simulink model "Power_Generator_Working"  (R2019b)
settings: Solver=ode23tb  StartTime=0.0  StopTime=inf  RelTol=5e-3
model workspace (MAT data in the model file):
  PLC_IP_Address = 'localhost'
libraries: dspnetwork x28, powerlib x8, sps_avr x7, simulink x3, dspstat3 x2
Description:
  | Copyright 2008-2019 The MathWorks, Inc.
settings Model: FPTRunName=Active  EnablePacing=on  PacingRate=0.100000  ExtModeTrigMode=oneshot  ExtModeArmWhenConnect=off  ExtModeAutoUpdateStatusClock=off  Creator=MathWorks  LastModifiedBy=Barata
settings SolverCC: ZeroCrossAlgorithm=Adaptive
settings DataIOCC: SaveFormat=Array  SignalLoggingSaveFormat=ModelDataLogs  ReturnWorkspaceOutputs=off  SignalLoggingName=sigsOut  OutputTimes=[0:1/20:10]
settings OptimizationCC: BlockReduction=off  BooleanDataType=off  ExpressionDepthLimit=2147483647  InitFltsAndDblsToZero=on  EfficientMapNaN2IntZero=off  LifeSpan=inf
settings DebuggingCC: UnderspecifiedInitializationDetection=Classic  MergeDetectMultiDrivingBlocksExec=none  CheckExecutionContextPreStartOutputMsg=on  CheckExecutionContextRuntimeOutputMsg=on  SignalResolutionControl=TryResolveAllWithWarning  IgnoredZcDiagnostic=none  MultiTaskDSMMsg=warning  MultiTaskCondExecSysMsg=none  SigSpecEnsureSampleTimeMsg=none  FcnCallInpInsideContextMsg=warning  UnconnectedInputMsg=none  UnconnectedOutputMsg=none  UnconnectedLineMsg=none  StateNameClashWarn=warning  SFUnexpectedBacktrackingDiag=warning  SFNoUnconditionalDefaultTransitionDiag=warning  SFExecutionAtInitializationDiag=none  ArithmeticOperatorsInVariantConditions=warning
settings HardwareCC: ProdBitPerPointer=32  ProdBitPerSizeT=32  ProdBitPerPtrDiffT=32  ProdLargestAtomicFloat=None  ProdIntDivRoundTo=Undefined  ProdEndianess=Unspecified  ProdWordSize=32  ProdHWDeviceType=Specified  TargetUnknown=on
settings ModelReferenceCC: PropagateSignalLabelsOutOfModel=off
settings SFSimCC: SimUseLocalCustomCode=off  CustomCodeUndefinedFunction=UseInterfaceOnly
settings RTWCC: RTWUseLocalCustomCode=off
settings CodeAppCC: StateflowObjectComments=on
settings GRTTargetCC: TargetFcnLib=ansi_tfl_tmw.mat  TargetLangStandard=C89/C90 (ANSI)  GeneratePreprocessorConditionals=Disable all  CombineOutputUpdateFcns=off  GRTInterface=on
settings ConfigComp: CovMetricSettings=dw  CovHtmlReporting=on  CovSaveCumulativeToWorkspaceVar=on  CovSaveSingleToWorkspaceVar=on  CovExternalEMLEnable=off  CovSFcnEnable=off
settings SimscapeCC: SimscapeNormalizeSystem=off

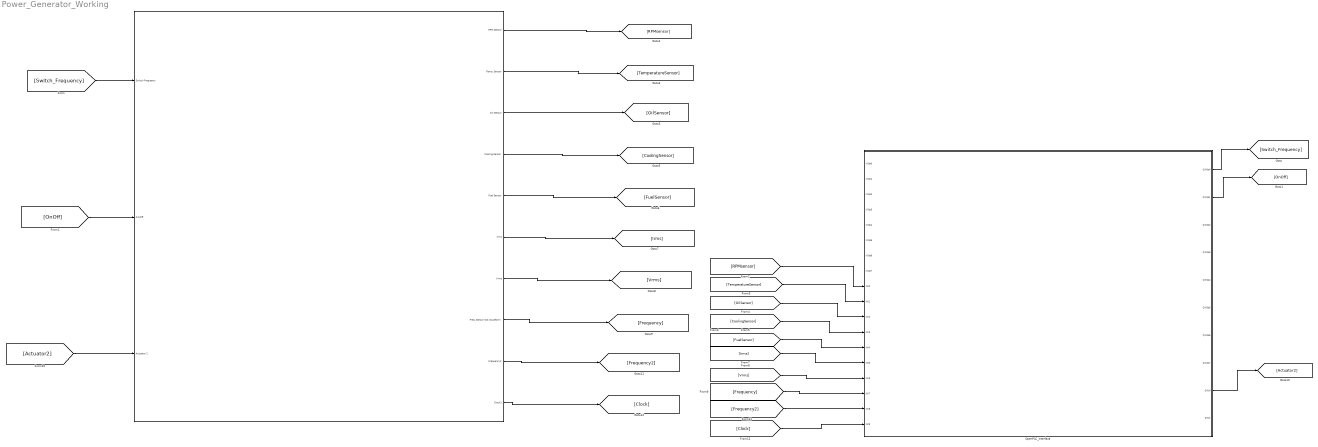
== system Power_Generator_Working ==
  " " : Subsystem
  OpenPLC_Interface : Subsystem
  wires:
  OpenPLC_Interface/2(QX0p1) -> [OnOff]
  [RPMsensor] -> OpenPLC_Interface/9(IW0)
  OpenPLC_Interface/1(QX0p0) -> [Switch_Frequency]
  [TemperatureSensor] -> OpenPLC_Interface/10(IW1)
  [OilSensor] -> OpenPLC_Interface/11(IW2)
  [CoolingSensor] -> OpenPLC_Interface/12(IW3)
  [FuelSensor] -> OpenPLC_Interface/13(IW4)
  [Irms] -> OpenPLC_Interface/14(IW5)
  [Vrms] -> OpenPLC_Interface/15(IW6)
  " "/1(RPM Sensor) -> [RPMsensor]
  " "/2("Temp. Sensor ") -> [TemperatureSensor]
  " "/4(Cooling Sensor) -> [CoolingSensor]
  " "/6(Irms) -> [Irms]
  " "/7(Vrms) -> [Vrms]
  " "/8("Freq. Sensor Not Waveform ") -> [Frequency]
  [Switch_Frequency] -> " "/1(Switch Frequency)
  [OnOff] -> " "/2(On/Off)
  [Frequency] -> OpenPLC_Interface/16(IW7)
  " "/3(Oil Sensor) -> [OilSensor]
  " "/5(Fuel Sensor) -> [FuelSensor]
  [Actuator2] -> " "/3(Actuator 2)
  OpenPLC_Interface/9(QW0) -> [Actuator2]
  " "/9(" Frequency2") -> [Frequency2]
  [Frequency2] -> OpenPLC_Interface/17(IW8)
  " "/10(Clock1) -> [Clock]
  [Clock] -> OpenPLC_Interface/18(IW9)

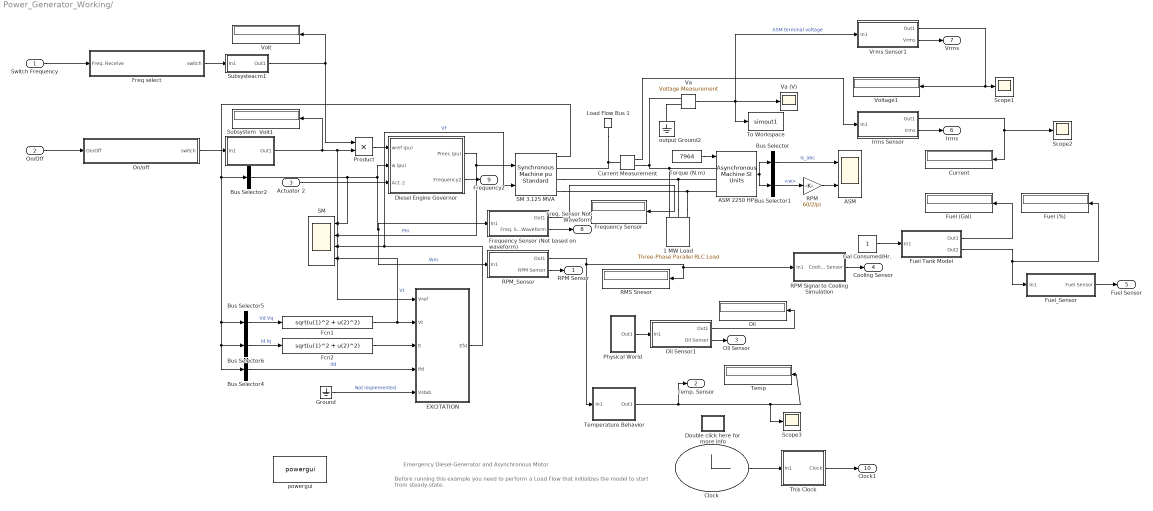
== system Power_Generator_Working/  ==
  note: Before running this example you need to perform a Load Flow that
      | initializes the model to start from steady-state.
  note: Emergency Diesel-Generator and Asynchronous Motor
  Switch Frequency : Inport
  On/Off : Inport  Port=2
  Actuator 2 : Inport  Port=3
  1 MW Load : powerlib/Elements/Three-Phase Parallel RLC Load  LConnTagsString=A|B|C  Configuration=Y (grounded)  NominalVoltage=2400  Vabc=[1e3 1e3 1e3]  Vabcp=[1e3 1e3 1e3]  NominalFrequency=60  UnbalancedPower=off  ActivePower=1e+006  InductivePower=0  CapacitivePower=0  Pabc=[10e3 9e3 11e3]  QLabc=[100 90 110]  QCabc=[100 90 110]  Pabcp=[10e3 9e3 11e3]  QLabcp=[100 90 110]  QCabcp=[100 90 110]  Measurements=None  LoadType=constant Z
      settings: SourceProductName=Simscape Electrical
  ASM : Scope  NumInputPorts=2
  ASM 2250 HP : powerlib/Machines/Asynchronous Machine SI Units  RotorType=Squirrel-cage  PresetModel=No  MechanicalLoad=Torque Tm  ShowDetailedParameters=on  ReferenceFrame=Rotor  Units=SI  MeasurementBus=on  NominalParameters=[ 2250*746, 2400, 60 ]  Stator=[ 0.029 0.226/377]  Rotor=[ 0.022 0.226/377]  Cage1=[ 0.022 0.226/377]  Cage2=[ 0.022 0.226/377]  Lm=13.04/377  Mechanical=[ 63.87 0 2]  PolePairs=2  InitialConditions=[0 0 0 0 0 0 0 0]  SimulateSaturation=off  Saturation=[14.03593122, 27.81365428, 53.79336849, 72.68890987, 97.98006896, 148.6815601, 215.7428561, 302.9841135, 428.7778367 ; 230, 322, 414, 460, 506, 552, 598, 644, 690]  LoadFlowParameters=1492000  TsPowergui=0  TsBlock=-1  IterativeModel=Trapezoidal non iterative  IterativeDiscreteModel=Trapezoidal non iterative  Pmec=1.492e+006
      settings: SourceProductName=Simscape Electrical
  Bus Selector : BusSelector  OutputSignals=ias,ibs,ics  OutputAsBus=on
  Bus Selector1 : BusSelector  OutputSignals=w
  Bus Selector2 : BusSelector  OutputSignals="Mechanical.Rotor speed  wm  (pu)"  OutputAsBus=on
  Bus Selector4 : BusSelector  OutputSignals="dq0 components.Field current  ifd (pu)"  OutputAsBus=on
  Bus Selector5 : BusSelector  OutputSignals="dq0 components.Stator voltage  vd (pu),dq0 components.Stator voltage  vq (pu)"  OutputAsBus=on
  Bus Selector6 : BusSelector  OutputSignals="dq0 components.Stator current  id (pu),dq0 components.Stator current  iq (pu)"  OutputAsBus=on
  Clock : Clock
  Current : Display
  Current Measurement : powerlib/Measurements/Current Measurement  PhasorSimulation=off  OutputType=Complex  PSBequivalent=0
      settings: SourceProductName=Simscape Electrical
  Diesel Engine Governor : Subsystem  AncestorBlock=spsDieselMotorModel/Diesel Engine Governor  mask(Diesel Engine & Governor){K=40, Tr=[0.01 0.02 0.2], Ta=[0.25 0.009 0.0384], Tlim=[0 1.1], Td=0.024, Pm0=0}
      mask prompts: K "Regulator gain K:"; Tr "Regulator time constants [T1 T2 T3 ] (s) :"; Ta "Actuator time constants [T4 T5 T6] (s) :"; Tlim "Torque limits [Tmin Tmax] (pu) :"; Td "Engine time delay Td (s) :"; Pm0 "Initial value of mechanical power  Pm0 (pu) :"
      mask help:
      | This block implements a diesel engine and governor system. The first input is the reference speed and the second input is the measured speed. The output is the diesel engine mechanical power. The motor inertia should be combined with the generator inertia.
      |
      | The model consist of a regulator represented by the following transfer function:
      |
      |      Hc = K.(1+T3.s)/(1+T1.s+T1.T2.s^2)
      |
      | The trotte actuator is implemented as :
      |
      |      Ha =  (1+T4.s) / [ (s (1+T5.s)(1+T6.s) ]
      |
      | The motor engine is represented by a Time delay Td function.
      mask Help:
      | This block implements a diesel engine and governor system. The first input is the reference speed and the second input is the measured speed. The output is the diesel engine mechanical power. The motor inertia should be combined with the generator inertia.
      | 
      | The model consist of a regulator represented by the following transfer function:
      | 
      |      Hc = K.(1+T3.s)/(1+T1.s+T1.T2.s^2)
      | 
      | The trotte actuator is implemented as :
      | 
      |      Ha =  (1+T4.s) / [ (s (1+T5.s)(1+T6.s) ]
      | 
      | The motor engine is represented by a Time delay Td function.
  Double click here for more info : Subsystem
      settings: OpenFcn=showdemo(bdroot(gcb))
      mask Display: disp('?')
  EXCITATION : Subsystem  VariantControlMode=Label  Variant=on  LabelModeActiveChoice=Variant1
      settings: AttributesFormatString=%<BlockChoice>
  Fcn1 : Fcn  Expr=sqrt(u(1)^2 + u(2)^2)
  Fcn2 : Fcn  Expr=sqrt(u(1)^2 + u(2)^2)
  Freq select : Subsystem
  Frequency Sensor : Display
  Frequency Sensor (Not based on waveform) : Subsystem
  Fuel (%) : Display
  Fuel (Gal) : Display
  Fuel Tank Model : Subsystem
  Fuel_Sensor : Subsystem
  "Gal Consumed/Hr. " : Constant
  Ground : Ground
  Irms Sensor : Subsystem
  Load Flow Bus 1 : powerlib/Measurements/Load Flow Bus  LConnTagsString=a  Phases=single  Connectors=on one side  ID=B2  Vbase=2.4e3  Vref=1  Vangle=0  VLF=1  VLFb=1  VLFc=1  angleLF=-31.89  angleLFb=0  angleLFc=0
      settings: AttributesFormatString=%<ID>\n%<Vbase>V\n%<VLF>pu\n%<angleLF>deg.  SourceProductName=Simscape Electrical
  Oil : Display
  Oil Sensor1 : Subsystem
  On/off : Subsystem
  Physical World : Subsystem
  Product : Product
  RMS Snesor : Display
  RPM : Gain  Gain=60/2/pi  SaturateOnIntegerOverflow=on  OutDataTypeStr=Inherit: Same as input  ParamDataTypeStr=Inherit: Same as input
  RPM Signal to Cooling Simulation : Subsystem
  RPM_Sensor : Subsystem
  SM : Scope  NumInputPorts=4
  SM 3.125 MVA : powerlib/Machines/Synchronous Machine pu Standard  PresetModel=No  MechanicalLoad=Mechanical power Pm  ShowDetailedParameters=on  RotorType=Salient-pole  Units=per unit standard parameters  MeasurementBus=off  NominalParameters="[ 3.125e6  2400  60]"  Reactances1=[ 31 32 33 34 35 36 37 ]  Reactances2=[ 1.56, 0.296, 0.177, 1.06, 0.177, 0.052 ]  dAxisTimeConstants=Short-circuit  qAxisTimeConstants=Open-circuit  TimeConstants1=[]  TimeConstants2=[]  TimeConstants3=[]  TimeConstants4=[]  TimeConstants5=[ 3.7, 0.05, 0.05 ]  TimeConstants6=[ 8.0, 0.03, 0.3371, 0.0295 ]  TimeConstants7=[0.024 0.006 0.006]  TimeConstants8=[]  StatorResistance=0.0036  Mechanical="[ 1.07  0 2]"  PolePairs=2  InitialConditions=[0 0 0 0 0 0 0 0 1]  SetSaturation=off  Saturation=[0.211 0.418 1.0 1.25 1.72 3.35 ;0.25 0.50 1.0 1.1 1.2 1.4]  LoadFlowParameters=[1 0 0 0]  TsPowergui=0  TsBlock=-1  IterativeModel=Trapezoidal non iterative  IterativeDiscreteModel=Trapezoidal non iterative  BusType=PV  Pref=0  Qref=0  Qmin=-Inf  Qmax=Inf  PLF=0  QLF=0
      settings: AttributesFormatString=\n\n  SourceProductName=Simscape Electrical
  Scope1 : Scope
  Scope2 : Scope
  Scope3 : Scope
  Subsysteacm1 : Subsystem
  Subsystem : Subsystem
  Temp : Display
  Temperature Behavior : Subsystem
  This Clock : Subsystem
  To Workspace : ToWorkspace  VariableName=simout1  SaveFormat=Timeseries  SampleTime=-1
  Torque (N.m) : Constant  Value=7964
  Va : powerlib/Measurements/Voltage Measurement  Tag=PoWeRsYsTeMmEaSuReMeNt  PhasorSimulation=off  OutputType=Magnitude  PSBequivalent=0
      settings: SourceProductName=Simscape Electrical
  Va (V) : Scope
  Volt : Display
  Volt1 : Display
  Voltage1 : Display
  Vrms Sensor1 : Subsystem
  output Ground2 : powerlib/Elements/Ground  LConnTagsString=a
      settings: SourceProductName=Simscape Electrical
  powergui : powerlib/powergui  Priority=2  SimulationMode=Discrete  SampleTime=100e-6  frequency=60  Iterations=50  frequencyindice=60  Pbase=1e6  ErrMax=0.0001  UnitsV=kV  UnitsW=MW  buscounter=0  FunctionMessages=off  echomessages=off  EnableUseOfTLC=off  CurrentSourceSwitches=off  DisableSnubberDevices=on  DisableRonSwitches=off  DisableVfSwitches=off  DisplayEquations=off  AutomaticDiscreteSolvers=off  SolverType=Tustin  Interpol=off  ExternalGateDelay=off  methode=off  Ts=0  x0status=blocks  SPID=on  SwTol=0  HookPort=off  NonlinearTolerance=0  nMaxIteration=15  ContinueOnMaxIteration=off  RestoreLinks=warning  ResistiveCurrentMeasurement=off  Frange=logspace(0,3,50)  Ylog=off  Xlog=off  ShowGrid=off  save=off  variable=ZData  structure=0  ZoomFFT=on  StartTime=0.0  cycles=2  DisplayStyle=off  fundamental=60  FreqAxis=off  MaxFrequency=1000  frequencyindicesteady=1  RmsSteady=1  display=off
      settings: SourceProductName=Simscape Electrical
  RPM Sensor : Outport  VectorParamsAs1DForOutWhenUnconnected=off
  "Temp. Sensor " : Outport  Port=2
  Oil Sensor : Outport  Port=3
  Cooling Sensor : Outport  Port=4
  Fuel Sensor : Outport  Port=5
  Irms : Outport  Port=6
  Vrms : Outport  Port=7
  "Freq. Sensor Not Waveform " : Outport  Port=8  VectorParamsAs1DForOutWhenUnconnected=off
  " Frequency2" : Outport  Port=9  VectorParamsAs1DForOutWhenUnconnected=off
  Clock1 : Outport  Port=10
  wires:
  Vrms Sensor1/2(Vrms) -> Vrms/1
  Irms Sensor/2(Irms) -> Irms/1
  Fuel_Sensor/1(Fuel Sensor) -> Fuel Sensor/1
  RPM Signal to Cooling Simulation/1(Cooling Sensor) -> Cooling Sensor/1
  Oil Sensor1/2(Oil Sensor) -> Oil Sensor/1
  RPM_Sensor/2(RPM Sensor) -> RPM Sensor/1
  On/Off/1 -> On/off/1(On/Off)
  Switch Frequency/1 -> Freq select/1(Freq. Receive)
  Clock/1 -> This Clock/1(In1)
  RPM_Sensor/1(Out1) -> RPM Signal to Cooling Simulation/1(In1), RMS Snesor/1, Temperature Behavior/1(In1)
  Subsystem/1(Out1) -> Volt1/1, Product/2, EXCITATION/1(Vref)
  Vrms Sensor1/1(Out1) -> Voltage1/1, Scope1/1
  Product/1 -> Diesel Engine Governor/1(wref (pu))
  Fuel Tank Model/1(Out1) -> Fuel (Gal)/1
  "Gal Consumed/Hr. "/1 -> Fuel Tank Model/1(In1)
  Subsysteacm1/1(Out1) -> Volt/1, Product/1
  Frequency Sensor (Not based on waveform)/1(Out1) -> Frequency Sensor/1
  Physical World/1(Out1) -> Oil Sensor1/1(In1)
  Current Measurement/1 -> Irms Sensor/1(In1)
  Ground/1 -> EXCITATION/5(Vstab)  "Not implemented"
  Diesel Engine Governor/1(Pmec (pu)) -> SM 3.125 MVA/1, SM/2  "Pm"
  On/off/1("switch ") -> Subsystem/1(In1)
  Oil Sensor1/1(Out1) -> Oil/1
  Bus Selector2/1 -> SM/1, Diesel Engine Governor/2(w (pu)), Frequency Sensor (Not based on waveform)/1(In1), RPM_Sensor/1(In1)  "Wm"
  Fcn2/1 -> EXCITATION/3(It)
  Bus Selector/1 -> ASM/1  "Is_abc"
  Freq select/1("switch ") -> Subsysteacm1/1(In1)
  Bus Selector4/1 -> EXCITATION/4(Ifd)  "Ifd"
  Temperature Behavior/1(Out1) -> Temp/1, Scope3/1, "Temp. Sensor "/1
  Fcn1/1 -> EXCITATION/2(Vt), SM/4  "Vt"
  EXCITATION/1(Efd) -> SM 3.125 MVA/2, SM/3  "Vf"
  Bus Selector6/1 -> Fcn2/1  "Id Iq"
  Irms Sensor/1(Out1) -> Scope2/1, Current/1
  Bus Selector5/1 -> Fcn1/1  "Vd Vq"
  Va/1 -> Va (V)/1, Vrms Sensor1/1(In1), To Workspace/1  "ASM terminal voltage"
  SM 3.125 MVA/1 -> Bus Selector4/1, Bus Selector6/1, Bus Selector5/1, Bus Selector2/1
  Torque (N.m)/1 -> ASM 2250 HP/1
  ASM 2250 HP/1 -> Bus Selector1/1, Bus Selector/1
  Fuel Tank Model/2(Out2) -> Fuel (%)/1, Fuel_Sensor/1(In1)
  Bus Selector1/1 -> RPM/1  "<w>"
  RPM/1 -> ASM/2
  Frequency Sensor (Not based on waveform)/2("Freq. Sensor Not Waveform ") -> "Freq. Sensor Not Waveform "/1
  Actuator 2/1 -> Diesel Engine Governor/3(Act. 2)
  Diesel Engine Governor/2(Frequency2) -> " Frequency2"/1
  This Clock/1(Clock) -> Clock1/1
  connections:
  output Ground2/LConn1 -- Va/LConn2
  1 MW Load/LConn3 -- ASM 2250 HP/LConn3 -- SM 3.125 MVA/RConn3
  1 MW Load/LConn1 -- Va/LConn1 -- Current Measurement/RConn1 -- ASM 2250 HP/LConn1
  1 MW Load/LConn2 -- ASM 2250 HP/LConn2 -- SM 3.125 MVA/RConn2
  Current Measurement/LConn1 -- SM 3.125 MVA/RConn1 -- Load Flow Bus 1/LConn1

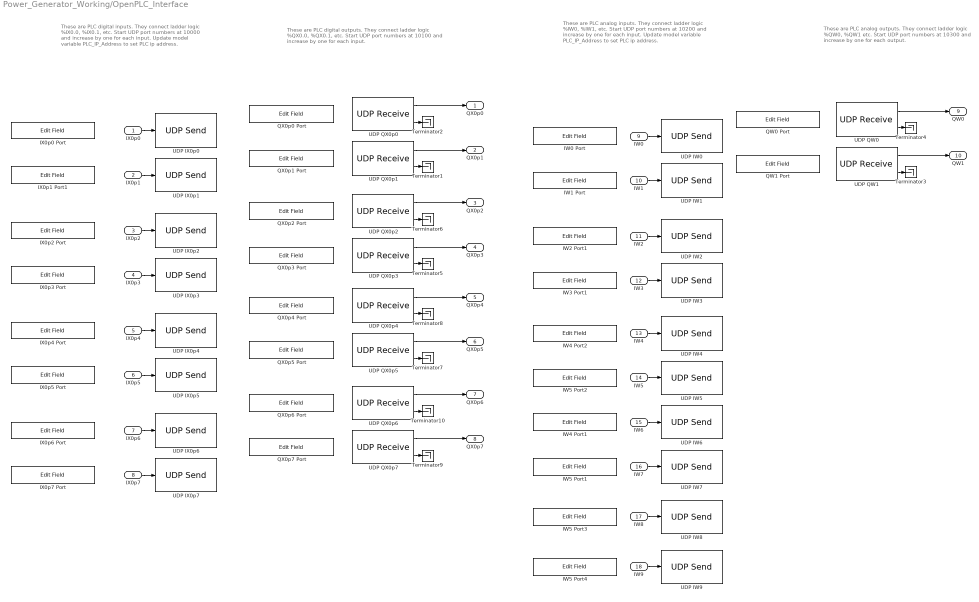
== system Power_Generator_Working/OpenPLC_Interface ==
  note: These are PLC digital inputs. They connect
      | ladder logic %IX0.0, %IX0.1, etc.
      |
      | Start UDP port numbers at 10000 and
      | increase by one for each input.
      |
      | Update model variable PLC_IP_Address
      | to set PLC ip address.
  note: These are PLC digital outputs. They connect
      | ladder logic %QX0.0, %QX0.1, etc.
      |
      | Start UDP port numbers at 10100 and increase
      | by one for each input.
  note: These are PLC analog inputs. They connect
      | ladder logic %IW0, %IW1, etc.
      |
      | Start UDP port numbers  at 10200 and
      | increase by one for each input.
      |
      | Update model variable PLC_IP_Address
      | to set PLC ip address.
  note: These are PLC analog outputs. They connect
      | ladder logic %QW0, %QW1 etc.
      |
      | Start UDP port numbers at 10300 and increase
      | by one for each output.
  "IX0p0 " : Inport
  IX0p1 : Inport  Port=2
  IX0p2 : Inport  Port=3
  IX0p3 : Inport  Port=4
  IX0p4 : Inport  Port=5
  IX0p5 : Inport  Port=6
  IX0p6 : Inport  Port=7
  IX0p7 : Inport  Port=8
  IW0 : Inport  Port=9
  IW1 : Inport  Port=10
  IW2 : Inport  Port=11
  IW3 : Inport  Port=12
  IW4 : Inport  Port=13
  IW5 : Inport  Port=14
  IW6 : Inport  Port=15
  IW7 : Inport  Port=16
  IW8 : Inport  Port=17
  IW9 : Inport  Port=18
  IW0 Port : EditField  LabelPosition=Hide  ShowInitialText=on  Alignment=Center
  IW1 Port : EditField  LabelPosition=Hide  ShowInitialText=on  Alignment=Center
  IW2 Port1 : EditField  LabelPosition=Hide  ShowInitialText=on  Alignment=Center
  IW3 Port1 : EditField  LabelPosition=Hide  ShowInitialText=on  Alignment=Center
  IW4 Port1 : EditField  LabelPosition=Hide  ShowInitialText=on  Alignment=Center
  IW4 Port2 : EditField  LabelPosition=Hide  ShowInitialText=on  Alignment=Center
  IW5 Port{1..4} (4 alike) : EditField  LabelPosition=Hide  ShowInitialText=on  Alignment=Center
  IX0p0 Port : EditField  LabelPosition=Hide  ShowInitialText=on  Alignment=Center
  IX0p1 Port1 : EditField  LabelPosition=Hide  ShowInitialText=on  Alignment=Center
  IX0p2 Port : EditField  LabelPosition=Hide  ShowInitialText=on  Alignment=Center
  IX0p3 Port : EditField  LabelPosition=Hide  ShowInitialText=on  Alignment=Center
  IX0p4 Port : EditField  LabelPosition=Hide  ShowInitialText=on  Alignment=Center
  IX0p5 Port : EditField  LabelPosition=Hide  ShowInitialText=on  Alignment=Center
  IX0p6 Port : EditField  LabelPosition=Hide  ShowInitialText=on  Alignment=Center
  IX0p7 Port : EditField  LabelPosition=Hide  ShowInitialText=on  Alignment=Center
  QW0 Port : EditField  LabelPosition=Hide  ShowInitialText=on  Alignment=Center
  QW1 Port : EditField  LabelPosition=Hide  ShowInitialText=on  Alignment=Center
  QX0p0 Port : EditField  LabelPosition=Hide  ShowInitialText=on  Alignment=Center
  QX0p1 Port : EditField  LabelPosition=Hide  ShowInitialText=on  Alignment=Center
  QX0p2 Port : EditField  LabelPosition=Hide  ShowInitialText=on  Alignment=Center
  QX0p3 Port : EditField  LabelPosition=Hide  ShowInitialText=on  Alignment=Center
  QX0p4 Port : EditField  LabelPosition=Hide  ShowInitialText=on  Alignment=Center
  QX0p5 Port : EditField  LabelPosition=Hide  ShowInitialText=on  Alignment=Center
  QX0p6 Port : EditField  LabelPosition=Hide  ShowInitialText=on  Alignment=Center
  QX0p7 Port : EditField  LabelPosition=Hide  ShowInitialText=on  Alignment=Center
  Terminator{1..10} (10 alike) : Terminator
  UDP IW0 : dspnetwork/UDP Send  remoteURL=PLC_IP_Address  remotePort=10200  localURL='255.255.255.255'  localPortSource=Automatically determine  localPort=-1  sampletime=-1  blockPlatform=LINUX  separateLengthPort=0
      settings: SourceProductName=DSP System Toolbox  SourceProductBaseCode=DS
  UDP IW1 : dspnetwork/UDP Send  remoteURL=PLC_IP_Address  remotePort=10201  localURL='255.255.255.255'  localPortSource=Automatically determine  localPort=-1  sampletime=-1  blockPlatform=LINUX  separateLengthPort=0
      settings: SourceProductName=DSP System Toolbox  SourceProductBaseCode=DS
  UDP IW2 : dspnetwork/UDP Send  remoteURL=PLC_IP_Address  remotePort=10202  localURL='255.255.255.255'  localPortSource=Automatically determine  localPort=-1  sampletime=-1  blockPlatform=LINUX  separateLengthPort=0
      settings: SourceProductName=DSP System Toolbox  SourceProductBaseCode=DS
  UDP IW3 : dspnetwork/UDP Send  remoteURL=PLC_IP_Address  remotePort=10203  localURL='255.255.255.255'  localPortSource=Automatically determine  localPort=-1  sampletime=-1  blockPlatform=LINUX  separateLengthPort=0
      settings: SourceProductName=DSP System Toolbox  SourceProductBaseCode=DS
  UDP IW4 : dspnetwork/UDP Send  remoteURL=PLC_IP_Address  remotePort=10204  localURL='255.255.255.255'  localPortSource=Automatically determine  localPort=-1  sampletime=-1  blockPlatform=LINUX  separateLengthPort=0
      settings: SourceProductName=DSP System Toolbox  SourceProductBaseCode=DS
  UDP IW5 : dspnetwork/UDP Send  remoteURL=PLC_IP_Address  remotePort=10205  localURL='255.255.255.255'  localPortSource=Automatically determine  localPort=-1  sampletime=-1  blockPlatform=LINUX  separateLengthPort=0
      settings: SourceProductName=DSP System Toolbox  SourceProductBaseCode=DS
  UDP IW6 : dspnetwork/UDP Send  remoteURL=PLC_IP_Address  remotePort=10206  localURL='255.255.255.255'  localPortSource=Automatically determine  localPort=-1  sampletime=-1  blockPlatform=LINUX  separateLengthPort=0
      settings: SourceProductName=DSP System Toolbox  SourceProductBaseCode=DS
  UDP IW7 : dspnetwork/UDP Send  remoteURL=PLC_IP_Address  remotePort=10207  localURL='255.255.255.255'  localPortSource=Automatically determine  localPort=-1  sampletime=-1  blockPlatform=LINUX  separateLengthPort=0
      settings: SourceProductName=DSP System Toolbox  SourceProductBaseCode=DS
  UDP IW8 : dspnetwork/UDP Send  remoteURL=PLC_IP_Address  remotePort=10208  localURL='255.255.255.255'  localPortSource=Automatically determine  localPort=-1  sampletime=-1  blockPlatform=LINUX  separateLengthPort=0
      settings: SourceProductName=DSP System Toolbox  SourceProductBaseCode=DS
  UDP IW9 : dspnetwork/UDP Send  remoteURL=PLC_IP_Address  remotePort=10209  localURL='255.255.255.255'  localPortSource=Automatically determine  localPort=-1  sampletime=-1  blockPlatform=LINUX  separateLengthPort=0
      settings: SourceProductName=DSP System Toolbox  SourceProductBaseCode=DS
  UDP IX0p0 : dspnetwork/UDP Send  remoteURL=PLC_IP_Address  remotePort=10000  localURL='255.255.255.255'  localPortSource=Automatically determine  localPort=-1  sampletime=-1  blockPlatform=LINUX  separateLengthPort=0
      settings: SourceProductName=DSP System Toolbox  SourceProductBaseCode=DS
  UDP IX0p1 : dspnetwork/UDP Send  remoteURL=PLC_IP_Address  remotePort=10001  localURL='255.255.255.255'  localPortSource=Automatically determine  localPort=-1  sampletime=-1  blockPlatform=LINUX  separateLengthPort=0
      settings: SourceProductName=DSP System Toolbox  SourceProductBaseCode=DS
  UDP IX0p2 : dspnetwork/UDP Send  remoteURL=PLC_IP_Address  remotePort=10002  localURL='255.255.255.255'  localPortSource=Automatically determine  localPort=-1  sampletime=-1  blockPlatform=LINUX  separateLengthPort=0
      settings: SourceProductName=DSP System Toolbox  SourceProductBaseCode=DS
  UDP IX0p3 : dspnetwork/UDP Send  remoteURL=PLC_IP_Address  remotePort=10003  localURL='255.255.255.255'  localPortSource=Automatically determine  localPort=-1  sampletime=-1  blockPlatform=LINUX  separateLengthPort=0
      settings: SourceProductName=DSP System Toolbox  SourceProductBaseCode=DS
  UDP IX0p4 : dspnetwork/UDP Send  remoteURL=PLC_IP_Address  remotePort=10004  localURL='255.255.255.255'  localPortSource=Automatically determine  localPort=-1  sampletime=-1  blockPlatform=LINUX  separateLengthPort=0
      settings: SourceProductName=DSP System Toolbox  SourceProductBaseCode=DS
  UDP IX0p5 : dspnetwork/UDP Send  remoteURL=PLC_IP_Address  remotePort=10005  localURL='255.255.255.255'  localPortSource=Automatically determine  localPort=-1  sampletime=-1  blockPlatform=LINUX  separateLengthPort=0
      settings: SourceProductName=DSP System Toolbox  SourceProductBaseCode=DS
  UDP IX0p6 : dspnetwork/UDP Send  remoteURL=PLC_IP_Address  remotePort=10006  localURL='255.255.255.255'  localPortSource=Automatically determine  localPort=-1  sampletime=-1  blockPlatform=LINUX  separateLengthPort=0
      settings: SourceProductName=DSP System Toolbox  SourceProductBaseCode=DS
  UDP IX0p7 : dspnetwork/UDP Send  remoteURL=PLC_IP_Address  remotePort=10007  localURL='255.255.255.255'  localPortSource=Automatically determine  localPort=-1  sampletime=-1  blockPlatform=LINUX  separateLengthPort=0
      settings: SourceProductName=DSP System Toolbox  SourceProductBaseCode=DS
  UDP QW0 : dspnetwork/UDP Receive  localURL='0.0.0.0'  localPort=10300  remoteURL='0.0.0.0'  remotePort=-1  recvBufferSize=2  dims=1  signalDatatype=uint16  isComplex=off  isVarSize=off  showBlockingTime=on  blockingTime=0  sampletime=0.01  blockPlatform=LINUX
      settings: SourceProductName=DSP System Toolbox  SourceProductBaseCode=DS
  UDP QW1 : dspnetwork/UDP Receive  localURL='0.0.0.0'  localPort=10301  remoteURL='0.0.0.0'  remotePort=-1  recvBufferSize=2  dims=1  signalDatatype=uint16  isComplex=off  isVarSize=off  showBlockingTime=on  blockingTime=0  sampletime=0.01  blockPlatform=LINUX
      settings: SourceProductName=DSP System Toolbox  SourceProductBaseCode=DS
  UDP QX0p0 : dspnetwork/UDP Receive  localURL='0.0.0.0'  localPort=10100  remoteURL='0.0.0.0'  remotePort=-1  recvBufferSize=2  dims=1  signalDatatype=uint16  isComplex=off  isVarSize=off  showBlockingTime=on  blockingTime=0  sampletime=0.01  blockPlatform=LINUX
      settings: SourceProductName=DSP System Toolbox  SourceProductBaseCode=DS
  UDP QX0p1 : dspnetwork/UDP Receive  localURL='0.0.0.0'  localPort=10101  remoteURL='0.0.0.0'  remotePort=-1  recvBufferSize=2  dims=1  signalDatatype=uint16  isComplex=off  isVarSize=off  showBlockingTime=on  blockingTime=0  sampletime=0.01  blockPlatform=LINUX
      settings: SourceProductName=DSP System Toolbox  SourceProductBaseCode=DS
  UDP QX0p2 : dspnetwork/UDP Receive  localURL='0.0.0.0'  localPort=10102  remoteURL='0.0.0.0'  remotePort=-1  recvBufferSize=2  dims=1  signalDatatype=uint16  isComplex=off  isVarSize=off  showBlockingTime=on  blockingTime=0  sampletime=0.01  blockPlatform=LINUX
      settings: SourceProductName=DSP System Toolbox  SourceProductBaseCode=DS
  UDP QX0p3 : dspnetwork/UDP Receive  localURL='0.0.0.0'  localPort=10103  remoteURL='0.0.0.0'  remotePort=-1  recvBufferSize=2  dims=1  signalDatatype=uint16  isComplex=off  isVarSize=off  showBlockingTime=on  blockingTime=0  sampletime=0.01  blockPlatform=LINUX
      settings: SourceProductName=DSP System Toolbox  SourceProductBaseCode=DS
  UDP QX0p4 : dspnetwork/UDP Receive  localURL='0.0.0.0'  localPort=10104  remoteURL='0.0.0.0'  remotePort=-1  recvBufferSize=2  dims=1  signalDatatype=uint16  isComplex=off  isVarSize=off  showBlockingTime=on  blockingTime=0  sampletime=0.01  blockPlatform=LINUX
      settings: SourceProductName=DSP System Toolbox  SourceProductBaseCode=DS
  UDP QX0p5 : dspnetwork/UDP Receive  localURL='0.0.0.0'  localPort=10105  remoteURL='0.0.0.0'  remotePort=-1  recvBufferSize=2  dims=1  signalDatatype=uint16  isComplex=off  isVarSize=off  showBlockingTime=on  blockingTime=0  sampletime=0.01  blockPlatform=LINUX
      settings: SourceProductName=DSP System Toolbox  SourceProductBaseCode=DS
  UDP QX0p6 : dspnetwork/UDP Receive  localURL='0.0.0.0'  localPort=10106  remoteURL='0.0.0.0'  remotePort=-1  recvBufferSize=2  dims=1  signalDatatype=uint16  isComplex=off  isVarSize=off  showBlockingTime=on  blockingTime=0  sampletime=0.01  blockPlatform=LINUX
      settings: SourceProductName=DSP System Toolbox  SourceProductBaseCode=DS
  UDP QX0p7 : dspnetwork/UDP Receive  localURL='0.0.0.0'  localPort=10107  remoteURL='0.0.0.0'  remotePort=-1  recvBufferSize=2  dims=1  signalDatatype=uint16  isComplex=off  isVarSize=off  showBlockingTime=on  blockingTime=0  sampletime=0.01  blockPlatform=LINUX
      settings: SourceProductName=DSP System Toolbox  SourceProductBaseCode=DS
  QX0p0 : Outport
  QX0p1 : Outport  Port=2
  QX0p2 : Outport  Port=3
  QX0p3 : Outport  Port=4
  QX0p4 : Outport  Port=5
  QX0p5 : Outport  Port=6
  QX0p6 : Outport  Port=7
  QX0p7 : Outport  Port=8
  QW0 : Outport  Port=9
  QW1 : Outport  Port=10
  wires:
  IX0p1/1 -> UDP IX0p1/1
  "IX0p0 "/1 -> UDP IX0p0/1
  UDP QX0p0/1 -> QX0p0/1
  UDP QX0p0/2 -> Terminator2/1
  UDP QX0p1/2 -> Terminator1/1
  UDP QX0p1/1 -> QX0p1/1
  IW1/1 -> UDP IW1/1
  IW0/1 -> UDP IW0/1
  UDP QW1/1 -> QW1/1
  UDP QW1/2 -> Terminator3/1
  UDP QW0/2 -> Terminator4/1
  UDP QW0/1 -> QW0/1
  IX0p2/1 -> UDP IX0p2/1
  IX0p3/1 -> UDP IX0p3/1
  IX0p7/1 -> UDP IX0p7/1
  IX0p6/1 -> UDP IX0p6/1
  IX0p4/1 -> UDP IX0p4/1
  IX0p5/1 -> UDP IX0p5/1
  UDP QX0p2/1 -> QX0p2/1
  UDP QX0p2/2 -> Terminator6/1
  UDP QX0p3/1 -> QX0p3/1
  UDP QX0p3/2 -> Terminator5/1
  UDP QX0p7/2 -> Terminator9/1
  UDP QX0p7/1 -> QX0p7/1
  UDP QX0p6/1 -> QX0p6/1
  UDP QX0p6/2 -> Terminator10/1
  UDP QX0p4/1 -> QX0p4/1
  UDP QX0p4/2 -> Terminator8/1
  UDP QX0p5/1 -> QX0p5/1
  UDP QX0p5/2 -> Terminator7/1
  IW3/1 -> UDP IW3/1
  IW2/1 -> UDP IW2/1
  IW5/1 -> UDP IW5/1
  IW4/1 -> UDP IW4/1
  IW7/1 -> UDP IW7/1
  IW6/1 -> UDP IW6/1
  IW8/1 -> UDP IW8/1
  IW9/1 -> UDP IW9/1

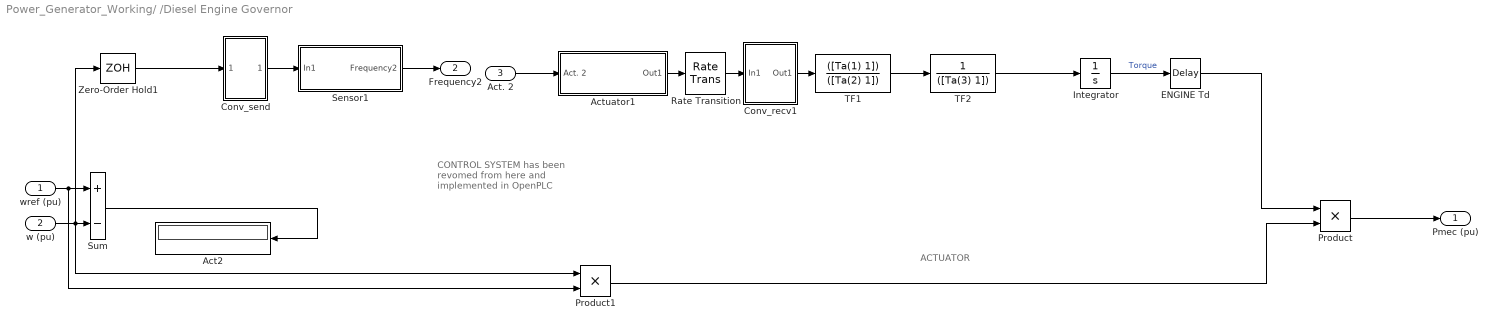
== system Power_Generator_Working/ /Diesel Engine Governor ==
  note: CONTROL SYSTEM
      | has been revomed from here
      | and implemented in
      | OpenPLC
  note: ACTUATOR
  wref (pu) : Inport
  w (pu) : Inport  Port=2
  Act. 2 : Inport  Port=3
  Act2 : Display
  Actuator1 : Subsystem
  Conv_recv1 : Subsystem
  Conv_send : Subsystem
  ENGINE Td : TransportDelay  DelayTime=Td  InitialOutput=Pm0
  Integrator : Integrator  InitialCondition=Pm0  LimitOutput=on  UpperSaturationLimit=Tlim(2)  LowerSaturationLimit=Tlim(1)
  Product : Product  SaturateOnIntegerOverflow=on  InputSameDT=on  OutDataTypeStr=Inherit: Same as first input
  Product1 : Product  SaturateOnIntegerOverflow=on  InputSameDT=on  OutDataTypeStr=Inherit: Same as first input
  Rate Transition : RateTransition
  Sensor1 : Subsystem
  Sum : Sum  Inputs=+-  SaturateOnIntegerOverflow=on  InputSameDT=on  OutDataTypeStr=Inherit: Same as first input
  TF1 : TransferFcn  Numerator=([Ta(1) 1])  Denominator=([Ta(2) 1])
  TF2 : TransferFcn  Numerator=1  Denominator=([Ta(3) 1])
  Zero-Order Hold1 : ZeroOrderHold  SampleTime=.02
  Pmec (pu) : Outport  InitialOutput=0  VectorParamsAs1DForOutWhenUnconnected=off
  Frequency2 : Outport  Port=2  VectorParamsAs1DForOutWhenUnconnected=off
  wires:
  Rate Transition/1 -> Conv_recv1/1(In1)
  Conv_send/1(Out1) -> Sensor1/1(In1)
  Conv_recv1/1(Out1) -> TF1/1
  Product1/1 -> Product/2
  Zero-Order Hold1/1 -> Conv_send/1(In1)
  Actuator1/1(Out1) -> Rate Transition/1
  Sum/1 -> Act2/1
  TF1/1 -> TF2/1
  w (pu)/1 -> Sum/2, Zero-Order Hold1/1, Product1/1
  ENGINE Td/1 -> Product/1
  wref (pu)/1 -> Sum/1, Product1/2
  Product/1 -> Pmec (pu)/1
  TF2/1 -> Integrator/1
  Integrator/1 -> ENGINE Td/1  "Torque"
  Act. 2/1 -> Actuator1/1(Act. 2)
  Sensor1/1("Frequency2 ") -> Frequency2/1

== system Power_Generator_Working/ /Double click here for more info ==

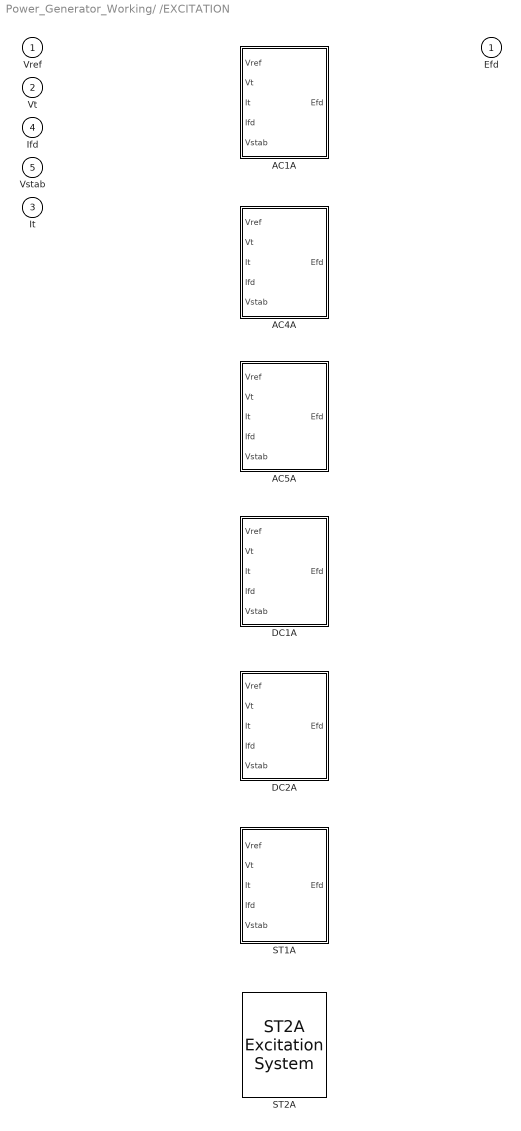
== system Power_Generator_Working/ /EXCITATION ==
  Vref : Inport
  Vt : Inport  Port=2
  It : Inport  Port=3
  Ifd : Inport  Port=4
  Vstab : Inport  Port=5
  AC1A : Subsystem  VariantControl=Variant1
  AC4A : Subsystem  VariantControl=Variant2
  AC5A : Subsystem  VariantControl=Variant3
  DC1A : Subsystem  VariantControl=Variant4
  DC2A : Subsystem  VariantControl=Variant5
  ST1A : Subsystem  VariantControl=Variant6
  ST2A : sps_avr/ST2A Excitation System  VariantControl=Variant7  Tr=20e-3  KaTa=[120 0.15]  VRminmax=[0 1.0]  KfTf=[0.05 1.0]  KeTe=[1.0 0.5]  KI=8.0  Kp=4.88  Xd=1.56  Kc=1.82  v0=[1,1.42734]  I0=0.2739  TsBlock=-2
      settings: SourceProductName=Simscape Electrical  SourceProductBaseCode=PS
  Efd : Outport  VectorParamsAs1DForOutWhenUnconnected=off

== system Power_Generator_Working/ /Freq select ==
  Freq. Receive : Inport
  Display : Display
  "switch " : Outport  PortDimensions=1  VectorParamsAs1DForOutWhenUnconnected=off
  wires:
  Freq. Receive/1 -> "switch "/1, Display/1

== system Power_Generator_Working/ /Frequency Sensor (Not based on waveform) ==
  In1 : Inport
  Downsample : DownSample  N=100  RateOptions=Allow multirate processing
  Gain : Gain  Gain=6000
  To Workspace1 : ToWorkspace  VariableName=Freq  SaveFormat=Timeseries  SampleTime=-1
  Zero-Order Hold : ZeroOrderHold  SampleTime=.001
  Out1 : Outport  VectorParamsAs1DForOutWhenUnconnected=off
  "Freq. Sensor Not Waveform " : Outport  Port=2  VectorParamsAs1DForOutWhenUnconnected=off
  wires:
  Gain/1 -> Downsample/1, To Workspace1/1
  Downsample/1 -> "Freq. Sensor Not Waveform "/1, Out1/1
  Zero-Order Hold/1 -> Gain/1
  In1/1 -> Zero-Order Hold/1

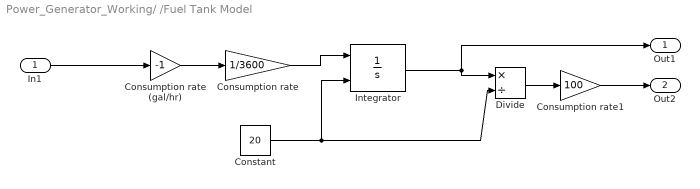
== system Power_Generator_Working/ /Fuel Tank Model ==
  In1 : Inport
  Constant : Constant  Value=20
  Consumption rate : Gain  Gain=1/3600
  Consumption rate (gal/hr) : Gain  Gain=-1
  Consumption rate1 : Gain  Gain=100
  Divide : Product  Inputs=*/
  Integrator : Integrator  InitialConditionSource=external  InitialCondition=20  LimitOutput=on  UpperSaturationLimit=20  LowerSaturationLimit=0
  Out1 : Outport  VectorParamsAs1DForOutWhenUnconnected=off
  Out2 : Outport  Port=2  VectorParamsAs1DForOutWhenUnconnected=off
  wires:
  Consumption rate/1 -> Integrator/1
  Consumption rate (gal/hr)/1 -> Consumption rate/1
  Divide/1 -> Consumption rate1/1
  Consumption rate1/1 -> Out2/1
  Integrator/1 -> Out1/1, Divide/1
  Constant/1 -> Integrator/2, Divide/2
  In1/1 -> Consumption rate (gal/hr)/1

== system Power_Generator_Working/ /Fuel_Sensor ==
  In1 : Inport
  Rate Transition : RateTransition
  To Workspace1 : ToWorkspace  VariableName=Fuel  SaveFormat=Timeseries  SampleTime=-1
  Zero-Order Hold : ZeroOrderHold  SampleTime=.001
  Zero-Order Hold1 : ZeroOrderHold  SampleTime=0.1
  Fuel Sensor : Outport
  wires:
  Zero-Order Hold1/1 -> Fuel Sensor/1
  Zero-Order Hold/1 -> To Workspace1/1
  In1/1 -> Zero-Order Hold/1, Rate Transition/1
  Rate Transition/1 -> Zero-Order Hold1/1

== system Power_Generator_Working/ /Irms Sensor ==
  In1 : Inport
  Downsample : DownSample  N=100  RateOptions=Allow multirate processing
  RMS : dspstat3/RMS  run=on  directionMode=Entire input  dimension=1  reset_popup=None
  To Workspace1 : ToWorkspace  VariableName=Current  SaveFormat=Timeseries  SampleTime=-1
  Zero-Order Hold : ZeroOrderHold  SampleTime=.001
  Out1 : Outport  VectorParamsAs1DForOutWhenUnconnected=off
  Irms : Outport  Port=2  VectorParamsAs1DForOutWhenUnconnected=off
  wires:
  Zero-Order Hold/1 -> RMS/1, To Workspace1/1
  Downsample/1 -> Irms/1, Out1/1
  RMS/1 -> Downsample/1
  In1/1 -> Zero-Order Hold/1

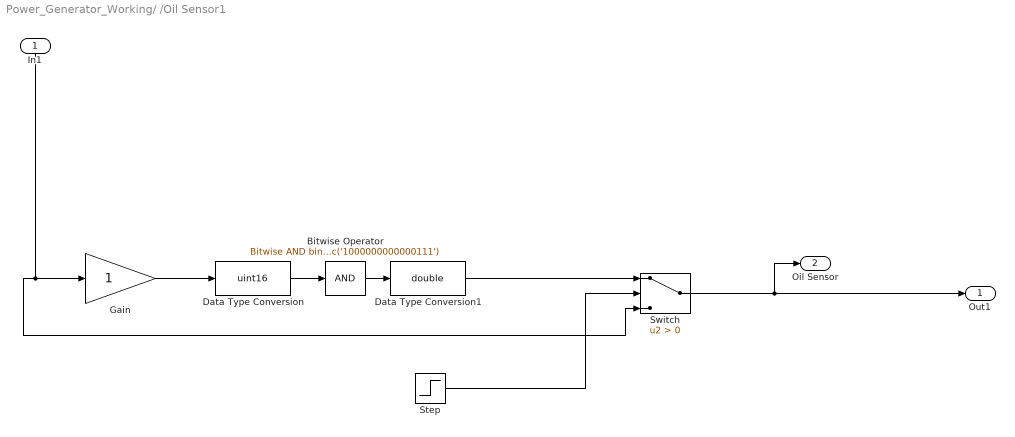
== system Power_Generator_Working/ /Oil Sensor1 ==
  In1 : Inport
  Bitwise Operator : simulink/Logic and Bit Operations/Bitwise Operator  logicop=AND  UseBitMask=on  BitMask=bin2dec('1000000000000111')  BitMaskRealWorld=Stored Integer
  Data Type Conversion : DataTypeConversion  OutDataTypeStr=uint16
  Data Type Conversion1 : DataTypeConversion  OutDataTypeStr=double
  Gain : Gain
  Step : Step  Time=200  SampleTime=0
  Switch : Switch  Criteria=u2 > Threshold
  Out1 : Outport  VectorParamsAs1DForOutWhenUnconnected=off
  Oil Sensor : Outport  Port=2  VectorParamsAs1DForOutWhenUnconnected=off
  wires:
  Step/1 -> Switch/2
  Data Type Conversion1/1 -> Switch/1
  Switch/1 -> Out1/1, Oil Sensor/1
  Data Type Conversion/1 -> Bitwise Operator/1
  Gain/1 -> Data Type Conversion/1
  Bitwise Operator/1 -> Data Type Conversion1/1
  In1/1 -> Switch/3, Gain/1

== system Power_Generator_Working/ /On//off ==
  On/Off : Inport
  Display : Display
  "switch " : Outport  PortDimensions=1  VectorParamsAs1DForOutWhenUnconnected=off
  wires:
  On/Off/1 -> Display/1, "switch "/1

== system Power_Generator_Working/ /Physical World ==
  Constant1 : Constant  Value=10
  Constant2 : Constant  Value=50
  Manual Switch : ManualSwitch
  Out1 : Outport  VectorParamsAs1DForOutWhenUnconnected=off
  wires:
  Manual Switch/1 -> Out1/1
  Constant1/1 -> Manual Switch/2
  Constant2/1 -> Manual Switch/1

== system Power_Generator_Working/ /RPM Signal to Cooling Simulation ==
  In1 : Inport
  Zero-Order Hold : ZeroOrderHold  SampleTime=.01
  Cooling Sensor : Outport  VectorParamsAs1DForOutWhenUnconnected=off
  wires:
  In1/1 -> Zero-Order Hold/1
  Zero-Order Hold/1 -> Cooling Sensor/1

== system Power_Generator_Working/ /RPM_Sensor ==
  In1 : Inport
  Downsample : DownSample  N=100  RateOptions=Allow multirate processing
  Gain : Gain  Gain=1800
  To Workspace : ToWorkspace  VariableName=RPM  SaveFormat=Timeseries  SampleTime=-1
  Zero-Order Hold : ZeroOrderHold  SampleTime=.001
  Out1 : Outport  VectorParamsAs1DForOutWhenUnconnected=off
  RPM Sensor : Outport  Port=2  VectorParamsAs1DForOutWhenUnconnected=off
  wires:
  Downsample/1 -> Out1/1, To Workspace/1, RPM Sensor/1
  Gain/1 -> Downsample/1
  Zero-Order Hold/1 -> Gain/1
  In1/1 -> Zero-Order Hold/1

== system Power_Generator_Working/ /Subsysteacm1 ==
  In1 : Inport
  Switch : Switch  Criteria=u2 > Threshold
  wref (pu) : Constant  Value=50/60
  wref (pu)1 : Constant
  Out1 : Outport  VectorParamsAs1DForOutWhenUnconnected=off
  wires:
  wref (pu)1/1 -> Switch/3
  Switch/1 -> Out1/1
  In1/1 -> Switch/2
  wref (pu)/1 -> Switch/1

== system Power_Generator_Working/ /Subsystem ==
  In1 : Inport
  Subtract : Sum  Inputs=+-
  "Vtref (pu) " : Constant
  Out1 : Outport  VectorParamsAs1DForOutWhenUnconnected=off
  wires:
  "Vtref (pu) "/1 -> Subtract/1
  In1/1 -> Subtract/2
  Subtract/1 -> Out1/1

== system Power_Generator_Working/ /Temperature Behavior ==
  In1 : Inport
  Exaust Temp Option : Subsystem
  Manual Switch : ManualSwitch
  Scope11 : Scope
  Temp : Subsystem
  Out1 : Outport  VectorParamsAs1DForOutWhenUnconnected=off
  wires:
  In1/1 -> Exaust Temp Option/1(In1), Temp/1(In1)
  Temp/1(Out1) -> Manual Switch/1
  Exaust Temp Option/1(Out1) -> Manual Switch/2, Scope11/1
  Manual Switch/1 -> Out1/1

== system Power_Generator_Working/ /This Clock ==
  In1 : Inport
  Zero-Order Hold : ZeroOrderHold
  Clock : Outport
  wires:
  In1/1 -> Zero-Order Hold/1
  Zero-Order Hold/1 -> Clock/1

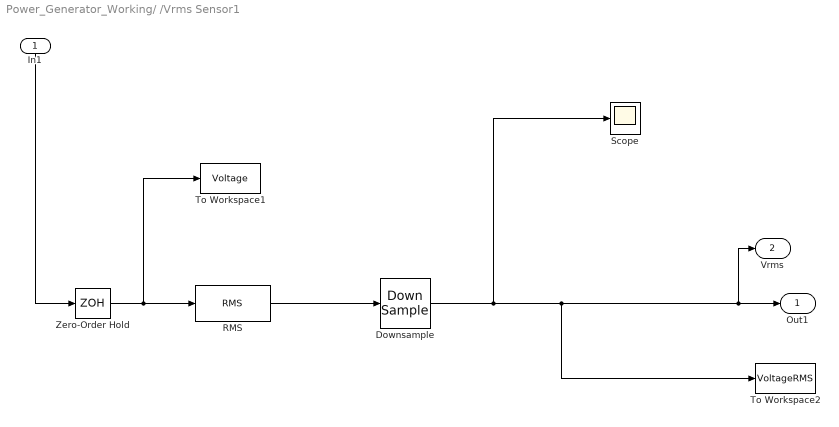
== system Power_Generator_Working/ /Vrms Sensor1 ==
  In1 : Inport
  Downsample : DownSample  N=100  RateOptions=Allow multirate processing
  RMS : dspstat3/RMS  run=on  directionMode=Entire input  dimension=1  reset_popup=None
  Scope : Scope
  To Workspace1 : ToWorkspace  VariableName=Voltage  SaveFormat=Timeseries  SampleTime=-1
  To Workspace2 : ToWorkspace  VariableName=VoltageRMS  SaveFormat=Timeseries  SampleTime=-1
  Zero-Order Hold : ZeroOrderHold  SampleTime=.001
  Out1 : Outport  VectorParamsAs1DForOutWhenUnconnected=off
  Vrms : Outport  Port=2  VectorParamsAs1DForOutWhenUnconnected=off
  wires:
  Zero-Order Hold/1 -> To Workspace1/1, RMS/1
  RMS/1 -> Downsample/1
  Downsample/1 -> Out1/1, Vrms/1, To Workspace2/1, Scope/1
  In1/1 -> Zero-Order Hold/1

== system Power_Generator_Working/ /Diesel Engine Governor/Actuator1 ==
  Act. 2 : Inport
  Voltage1 : Display
  Voltage2 : Display
  Out1 : Outport  VectorParamsAs1DForOutWhenUnconnected=off
  wires:
  Act. 2/1 -> Voltage1/1, Out1/1

== system Power_Generator_Working/ /Diesel Engine Governor/Conv_recv1 ==
  In1 : Inport
  Constant : Constant  Value=10000
  Constant1 : Constant  Value=1000
  Divide : Product  Inputs=*/
  Sum2 : Sum  Inputs=|+-
  Out1 : Outport  VectorParamsAs1DForOutWhenUnconnected=off
  wires:
  Constant1/1 -> Divide/2
  Constant/1 -> Sum2/2
  Sum2/1 -> Divide/1
  Divide/1 -> Out1/1
  In1/1 -> Sum2/1

== system Power_Generator_Working/ /Diesel Engine Governor/Conv_send ==
  In1 : Inport
  Constant : Constant  Value=1000
  Constant1 : Constant  Value=10000
  Product1 : Product
  Sum1 : Sum  Inputs=|++
  Out1 : Outport  VectorParamsAs1DForOutWhenUnconnected=off
  wires:
  Constant/1 -> Product1/2
  Constant1/1 -> Sum1/2
  Sum1/1 -> Out1/1
  In1/1 -> Product1/1
  Product1/1 -> Sum1/1

== system Power_Generator_Working/ /Diesel Engine Governor/Sensor1 ==
  In1 : Inport
  Scope : Scope
  To Workspace : ToWorkspace  VariableName=sen  SaveFormat=Timeseries  SampleTime=-1
  Zero-Order Hold : ZeroOrderHold  SampleTime=.01
  "Frequency2 " : Outport  VectorParamsAs1DForOutWhenUnconnected=off
  wires:
  Zero-Order Hold/1 -> "Frequency2 "/1, To Workspace/1, Scope/1
  In1/1 -> Zero-Order Hold/1

== system Power_Generator_Working/ /EXCITATION/AC1A ==
  Vref : Inport
  Vt : Inport  Port=2
  It : Inport  Port=3
  Ifd : Inport  Port=4
  Vstab : Inport  Port=5
  AC1A : sps_avr/AC1A Excitation System  Tr=20e-3  KaTa=[400 0.02]  VAminmax=[-14.5 14.5]  VRminmax=[-5.43 6.03]  KfTf=[0.03 1.0]  TbTc=[0 0]  KeTe=[1.0 0.80]  Ve12=[4.18 3.14]  SeVe12=[0.10 0.03]  Kd=0.38  Kc=0.20  v0=[1 1.4273]  TsBlock=-2
      settings: SourceProductName=Simscape Electrical  SourceProductBaseCode=PS
  term3 : Terminator
  Efd : Outport  VectorParamsAs1DForOutWhenUnconnected=off
  wires:
  Vref/1 -> AC1A/1
  Vt/1 -> AC1A/2
  Ifd/1 -> AC1A/3
  Vstab/1 -> AC1A/4
  AC1A/1 -> Efd/1
  It/1 -> term3/1

== system Power_Generator_Working/ /EXCITATION/AC4A ==
  Vref : Inport
  Vt : Inport  Port=2
  It : Inport  Port=3
  Ifd : Inport  Port=4
  Vstab : Inport  Port=5
  AC4A : sps_avr/AC4A Excitation System  Tr=20e-3  KaTa=[200 0.015]  VIminmax=[-10 10]  VRminmax=[-4.53 5.64]  TbTc=[10 1.0]  Kc=0  v0=[1,1.42734]  TsBlock=-2
      settings: SourceProductName=Simscape Electrical  SourceProductBaseCode=PS
  term3 : Terminator
  Efd : Outport  VectorParamsAs1DForOutWhenUnconnected=off
  wires:
  Vref/1 -> AC4A/1
  Vt/1 -> AC4A/2
  Ifd/1 -> AC4A/3
  Vstab/1 -> AC4A/4
  AC4A/1 -> Efd/1
  It/1 -> term3/1

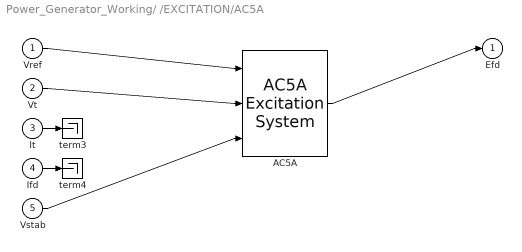
== system Power_Generator_Working/ /EXCITATION/AC5A ==
  Vref : Inport
  Vt : Inport  Port=2
  It : Inport  Port=3
  Ifd : Inport  Port=4
  Vstab : Inport  Port=5
  AC5A : sps_avr/AC5A Excitation System  Tr=20e-3  KaTa=[100 0.02]  VRminmax=[-7.3 7.3]  KfTf=[0.03 1 0 0]  KeTe=[1.0 0.02]  Efd12=[5.6 0.75*5.6]  SeEfd12=[0.86 0.5]  v0=[1,1.42734]  TsBlock=-2
      settings: SourceProductName=Simscape Electrical  SourceProductBaseCode=PS
  term3 : Terminator
  term4 : Terminator
  Efd : Outport  VectorParamsAs1DForOutWhenUnconnected=off
  wires:
  Vref/1 -> AC5A/1
  Vt/1 -> AC5A/2
  Vstab/1 -> AC5A/3
  AC5A/1 -> Efd/1
  It/1 -> term3/1
  Ifd/1 -> term4/1

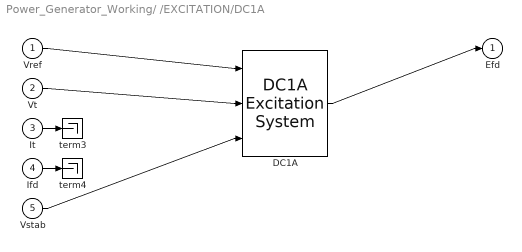
== system Power_Generator_Working/ /EXCITATION/DC1A ==
  Vref : Inport
  Vt : Inport  Port=2
  It : Inport  Port=3
  Ifd : Inport  Port=4
  Vstab : Inport  Port=5
  DC1A : sps_avr/DC1A Excitation System  Tr=20e-3  KaTa=[46 0.06]  VRminmax=[-0.9 1.0]  KfTf=[0.05 1.5]  TbTc=[0 0]  KeTe=[0.05 0.46]  Efd12=[3.1 2.3]  SeEfd12=[0.33 0.10]  v0=[1,1.42734]  TsBlock=-2
      settings: SourceProductName=Simscape Electrical  SourceProductBaseCode=PS
  term3 : Terminator
  term4 : Terminator
  Efd : Outport  VectorParamsAs1DForOutWhenUnconnected=off
  wires:
  Vref/1 -> DC1A/1
  Vt/1 -> DC1A/2
  Vstab/1 -> DC1A/3
  DC1A/1 -> Efd/1
  It/1 -> term3/1
  Ifd/1 -> term4/1

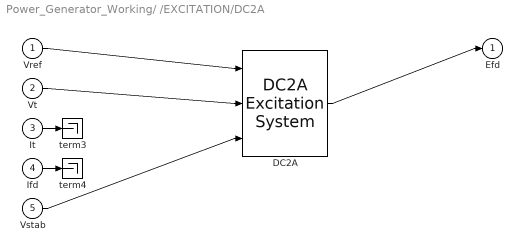
== system Power_Generator_Working/ /EXCITATION/DC2A ==
  Vref : Inport
  Vt : Inport  Port=2
  It : Inport  Port=3
  Ifd : Inport  Port=4
  Vstab : Inport  Port=5
  DC2A : sps_avr/DC2A Excitation System  Tr=20e-3  KaTa=[46 0.06]  VRminmax=[-4.9 4.95]  KfTf=[0.05 1.5]  TbTc=[0 0]  KeTe=[0.05 0.46]  Efd12=[3.05 2.29]  SeEfd12=[0.279 0.117]  v0=[1,1.42734]  TsBlock=-2
      settings: SourceProductName=Simscape Electrical  SourceProductBaseCode=PS
  term3 : Terminator
  term4 : Terminator
  Efd : Outport  VectorParamsAs1DForOutWhenUnconnected=off
  wires:
  Vref/1 -> DC2A/1
  Vt/1 -> DC2A/2
  Vstab/1 -> DC2A/3
  DC2A/1 -> Efd/1
  It/1 -> term3/1
  Ifd/1 -> term4/1

== system Power_Generator_Working/ /EXCITATION/ST1A ==
  Vref : Inport
  Vt : Inport  Port=2
  It : Inport  Port=3
  Ifd : Inport  Port=4
  Vstab : Inport  Port=5
  ST1A : sps_avr/ST1A Excitation System  Tr=20e-3  KaTa=[210 0.001]  VIminmax=[-999 999]  VAminmax=[-999 999]  VRminmax=[-6.0 6.43]  KfTf=[0.001 1]  TbTc=[0 0 0 0]  KLR=1  ILR=2  Kc=0.038  v0=[1,1.42734]  TsBlock=-2
      settings: SourceProductName=Simscape Electrical  SourceProductBaseCode=PS
  term3 : Terminator
  Efd : Outport  VectorParamsAs1DForOutWhenUnconnected=off
  wires:
  Vref/1 -> ST1A/1
  Vt/1 -> ST1A/2
  Ifd/1 -> ST1A/3
  Vstab/1 -> ST1A/4
  ST1A/1 -> Efd/1
  It/1 -> term3/1

== system Power_Generator_Working/ /Temperature Behavior/Exaust Temp Option ==
  In1 : Inport
  1-D Lookup Table3 : Lookup_n-D  NumberOfTableDimensions=1  BreakpointsForDimension1=[998.92,1036.7,1066.9,1099.6,1129.9,1160.1,1192.8,1223,1255.8,1286,1316.2,1348.9,1379.1,1409.4,1442.1,1469.8,1505,1535.3,1565.5,1598.2,1625.9,1658.6,1686.3,1714,1739.2,1769.4,1794.6,1824.8,1852.5,1877.7,1905.4,1928.1,1955.8,1980.9,2003.6]  Table=[124.82,125.06,125.3,125.77,126.25,126.96,127.91,128.62,129.8,130.99,131.94,133.6,135.02,136.68,138.58,140.47,142.61,144.27,146.64,149.01,151.38,153.99,156.36,158.74,161.11,163.95,166.56,169.64,172.49,175.34,178.42,181.03,184.11,187.19,189.09]  InternalRulePriority=Speed  RndMeth=Simplest  InputSameDT=on
  Add8 : Sum
  Band-Limited White Noise5 : simulink/Sources/Band-Limited White Noise  Cov=[0.001]  Ts=0.02  seed=[233]
  Scope10 : Scope
  Out1 : Outport  VectorParamsAs1DForOutWhenUnconnected=off
  wires:
  1-D Lookup Table3/1 -> Add8/1, Scope10/1
  Band-Limited White Noise5/1 -> Add8/2
  Add8/1 -> Out1/1
  In1/1 -> 1-D Lookup Table3/1

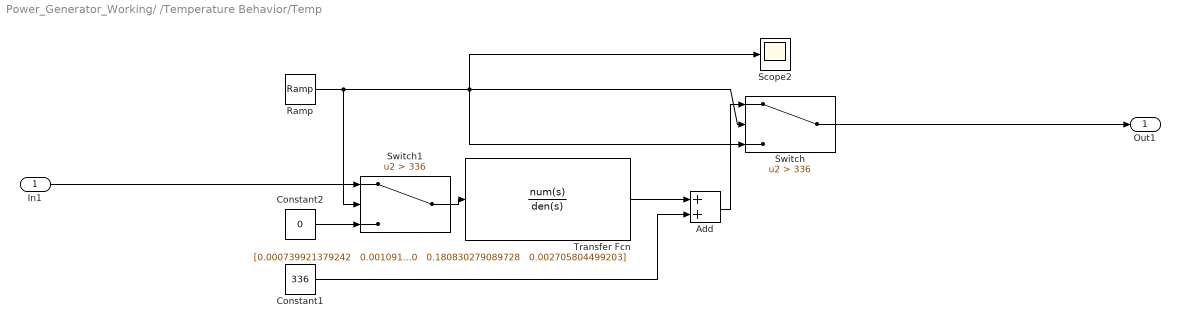
== system Power_Generator_Working/ /Temperature Behavior/Temp ==
  In1 : Inport
  Add : Sum
  Constant1 : Constant  Value=336
  Constant2 : Constant  Value=0
  Ramp : simulink/Sources/Ramp  slope=336/50  start=0  InitialOutput=0
  Scope2 : Scope
  Switch : Switch  Criteria=u2 > Threshold  Threshold=336
  Switch1 : Switch  Criteria=u2 > Threshold  Threshold=336
  Transfer Fcn : TransferFcn  Numerator="[0.000739921379242   0.001091115494706   0.000083546970890]"  Denominator="[1.000000000000000   0.180830279089728   0.002705804499203]"
  Out1 : Outport  VectorParamsAs1DForOutWhenUnconnected=off
  wires:
  Switch/1 -> Out1/1
  Constant1/1 -> Add/2
  In1/1 -> Switch1/1
  Switch1/1 -> Transfer Fcn/1
  Transfer Fcn/1 -> Add/1
  Ramp/1 -> Scope2/1, Switch/2, Switch/3, Switch1/2
  Constant2/1 -> Switch1/3
  Add/1 -> Switch/1
